simulink model "grid_test"  (R2013a)
settings: Solver=ode3  StartTime=0.0  StopTime=0.1  FixedStep=100e-6  RelTol=1e-3
undefined symbols (not defined in the file): Ts
libraries: powerlib x13, cables_lib x4, simulink x2, controllable_grid_lib x1, powerlib_extras x1
settings Model: Creator=pkoralew  LastModifiedBy=pkoralew

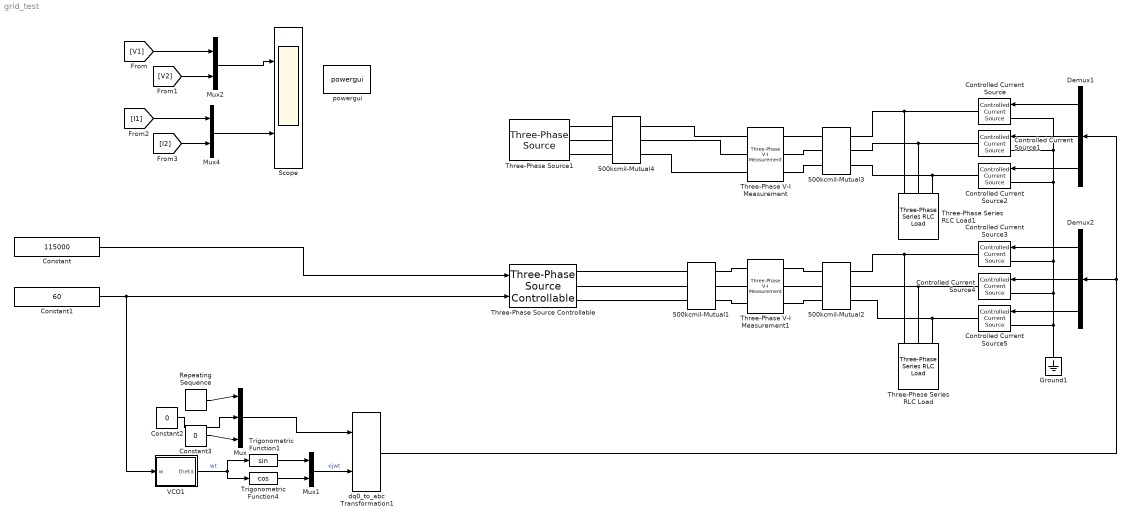
== system grid_test ==
  500kcmil-Mutual{1..4} (4 alike) : cables_lib/500kcmil-Mutual  length=50  par_sets=1  ratio=3
  Constant : Constant  Value=115000
  Constant1 : Constant  Value=60
  Constant2 : Constant  Value=0
  Constant3 : Constant  Value=0
  Controlled Current Source{,1..5} (6 alike) : powerlib/Electrical Sources/Controlled Current Source  Initialize=on  Source_Type=AC  Amplitude=0  Phase=0  Frequency=0  Measurements=None
  Demux1 : Demux  Outputs=3
  Demux2 : Demux  Outputs=3
  Ground1 : powerlib/Elements/Ground  LConnTagsString=a
  Mux : Mux  Inputs=3
  Mux1 : Mux  Inputs=2
  Mux2 : Mux  Inputs=2
  Mux4 : Mux  Inputs=2
  Repeating Sequence : simulink/Sources/Repeating Sequence  rep_seq_t=[0 0.05 0.0501 0.1]  rep_seq_y=[0 0 1000 1000]
  Scope : Scope  NumInputPorts=2
      settings: YMin=-5~-5  YMax=5~5
  Three-Phase Series RLC Load : powerlib/Elements/Three-Phase Series RLC Load  LConnTagsString=A|B|C  Configuration=Y (grounded)  NominalVoltage=115000  NominalFrequency=60  ActivePower=100e3  InductivePower=0  CapacitivePower=0  Measurements=None  LoadType=constant Z
  Three-Phase Series RLC Load1 : powerlib/Elements/Three-Phase Series RLC Load  LConnTagsString=A|B|C  Configuration=Y (grounded)  NominalVoltage=115000  NominalFrequency=60  ActivePower=100e3  InductivePower=0  CapacitivePower=0  Measurements=None  LoadType=constant Z
  Three-Phase V-I Measurement : powerlib/Measurements/Three-Phase V-I Measurement  VoltageMeasurement=phase-to-ground  SetLabelV=on  LabelV=V1  Vpu=off  VpuLL=off  CurrentMeasurement=yes  SetLabelI=on  LabelI=I1  Ipu=off  Pbase=100e6  Vbase=500e3  OutputType=Complex  PhasorSimulation=off  PSBequivalent=0
  Three-Phase V-I Measurement1 : powerlib/Measurements/Three-Phase V-I Measurement  VoltageMeasurement=phase-to-ground  SetLabelV=on  LabelV=V2  Vpu=off  VpuLL=off  CurrentMeasurement=yes  SetLabelI=on  LabelI=I2  Ipu=off  Pbase=100e6  Vbase=500e3  OutputType=Complex  PhasorSimulation=off  PSBequivalent=0
  Three-Phase Source Controllable : controllable_grid_lib/Three-Phase Source Controllable  mask{Ts=Ts}
  Three-Phase Source1 : powerlib/Electrical Sources/Three-Phase Source  Voltage=115000  PhaseAngle=0  Frequency=60  InternalConnection=Yg  SpecifyImpedance=on  Resistance=0.8929  Inductance=16.58e-3  ShortCircuitLevel=2000e6  BaseVoltage=115000  XRratio=100  BusType=swing  Pref=0  Qref=0  Qmin=-inf  Qmax=inf
  Trigonometric Function1 : Trigonometry
  Trigonometric Function4 : Trigonometry  Operator=cos
  VCO1 : Subsystem
  dq0_to_abc Transformation1 : powerlib_extras/Measurements/dq0_to_abc Transformation
  powergui : powerlib/powergui  Priority=1  SimulationMode=Discrete  SolverType=Tustin  SampleTime=100e-6  frequency=60  SPID=off  DisableSnubberDevices=off  DisableRonSwitches=off  DisableVfSwitches=off  SwTol=0  Interpol=off  DisplayEquations=off  frequencyindice=0  Pbase=100e6  ErrMax=1e-4  Iterations=50  UnitsV=kV  UnitsW=MW  FunctionMessages=off  echomessages=off  HookPort=off  EnableUseOfTLC=off  x0status=blocks  RestoreLinks=warning  ResistiveCurrentMeasurement=off  Frange=[0:2:500]  Ylog=off  Xlog=on  ShowGrid=off  save=off  variable=ZData  ZoomFFT=off  StartTime=0.0  cycles=1  DisplayStyle=1  fundamental=60  FreqAxis=off  MaxFrequency=1000  frequencyindicesteady=1  RmsSteady=1  display=off  Ts=0  methode=off
  wires:
  Mux1/1 -> dq0_to_abc Transformation1/2  "ejwt"
  VCO1/1(theta) -> Trigonometric Function4/1, Trigonometric Function1/1  "wt"
  Trigonometric Function1/1 -> Mux1/1
  Trigonometric Function4/1 -> Mux1/2
  Mux/1 -> dq0_to_abc Transformation1/1
  Constant1/1 -> Three-Phase Source Controllable/2, VCO1/1(w)
  Repeating Sequence/1 -> Mux/1
  Constant2/1 -> Mux/2
  Constant3/1 -> Mux/3
  Demux1/2 -> Controlled Current Source1/1
  Demux1/1 -> Controlled Current Source/1
  Demux1/3 -> Controlled Current Source2/1
  Demux2/1 -> Controlled Current Source3/1
  Demux2/2 -> Controlled Current Source4/1
  Demux2/3 -> Controlled Current Source5/1
  dq0_to_abc Transformation1/1 -> Demux2/1, Demux1/1
  Mux2/1 -> Scope/1
  Mux4/1 -> Scope/2
  [V1] -> Mux2/1
  [V2] -> Mux2/2
  [I1] -> Mux4/1
  [I2] -> Mux4/2
  Constant/1 -> Three-Phase Source Controllable/1
  connections:
  500kcmil-Mutual4/LConn2 -- Three-Phase Source1/RConn2
  500kcmil-Mutual4/LConn1 -- Three-Phase Source1/RConn1
  500kcmil-Mutual4/LConn3 -- Three-Phase Source1/RConn3
  Three-Phase V-I Measurement/LConn1 -- 500kcmil-Mutual4/RConn1
  Three-Phase V-I Measurement/LConn2 -- 500kcmil-Mutual4/RConn2
  Three-Phase V-I Measurement/LConn3 -- 500kcmil-Mutual4/RConn3
  500kcmil-Mutual1/RConn2 -- Three-Phase V-I Measurement1/LConn2
  500kcmil-Mutual1/RConn1 -- Three-Phase V-I Measurement1/LConn1
  500kcmil-Mutual1/RConn3 -- Three-Phase V-I Measurement1/LConn3
  Ground1/LConn1 -- Controlled Current Source5/LConn1 -- Controlled Current Source4/LConn1 -- Controlled Current Source3/LConn1 -- Controlled Current Source2/LConn1 -- Controlled Current Source1/LConn1 -- Controlled Current Source/LConn1
  Three-Phase V-I Measurement/RConn1 -- 500kcmil-Mutual3/LConn1
  Three-Phase V-I Measurement/RConn2 -- 500kcmil-Mutual3/LConn2
  Three-Phase V-I Measurement/RConn3 -- 500kcmil-Mutual3/LConn3
  Three-Phase V-I Measurement1/RConn2 -- 500kcmil-Mutual2/LConn2
  Three-Phase V-I Measurement1/RConn3 -- 500kcmil-Mutual2/LConn3
  Three-Phase V-I Measurement1/RConn1 -- 500kcmil-Mutual2/LConn1
  500kcmil-Mutual3/RConn1 -- Three-Phase Series RLC Load1/LConn1 -- Controlled Current Source/RConn1
  Controlled Current Source1/RConn1 -- Three-Phase Series RLC Load1/LConn2 -- 500kcmil-Mutual3/RConn2
  500kcmil-Mutual3/RConn3 -- Three-Phase Series RLC Load1/LConn3 -- Controlled Current Source2/RConn1
  Controlled Current Source3/RConn1 -- Three-Phase Series RLC Load/LConn1 -- 500kcmil-Mutual2/RConn1
  500kcmil-Mutual2/RConn2 -- Three-Phase Series RLC Load/LConn2 -- Controlled Current Source4/RConn1
  Controlled Current Source5/RConn1 -- Three-Phase Series RLC Load/LConn3 -- 500kcmil-Mutual2/RConn3
  Three-Phase Source Controllable/RConn1 -- 500kcmil-Mutual1/LConn1
  Three-Phase Source Controllable/RConn2 -- 500kcmil-Mutual1/LConn2
  Three-Phase Source Controllable/RConn3 -- 500kcmil-Mutual1/LConn3

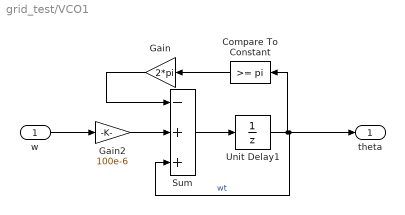
== system grid_test/VCO1 ==
  w : Inport
  Compare To Constant : simulink/Logic and Bit Operations/Compare To Constant  relop=>=  const=pi  OutDataTypeStr=uint8
  Gain : Gain  Gain=2*pi  OutDataTypeStr=double
  Gain2 : Gain  Gain=100e-6  SaturateOnIntegerOverflow=on  OutDataTypeStr=Inherit: Same as input  ParamDataTypeStr=Inherit: Same as input
  Sum : Sum  Inputs=-++
  Unit Delay1 : UnitDelay  SampleTime=-1
  theta : Outport
  wires:
  w/1 -> Gain2/1
  Gain/1 -> Sum/1
  Compare To Constant/1 -> Gain/1
  Unit Delay1/1 -> Compare To Constant/1, Sum/3, theta/1  "wt"
  Gain2/1 -> Sum/2
  Sum/1 -> Unit Delay1/1
